simulink model "pruebaswitch2"  (R2016b)
settings: Solver=VariableStepAuto  StartTime=0.0  StopTime=10.0  RelTol=1e-3
undefined symbols (not defined in the file): LD
settings Model: Creator=Uxío  LastModifiedBy=Uxío

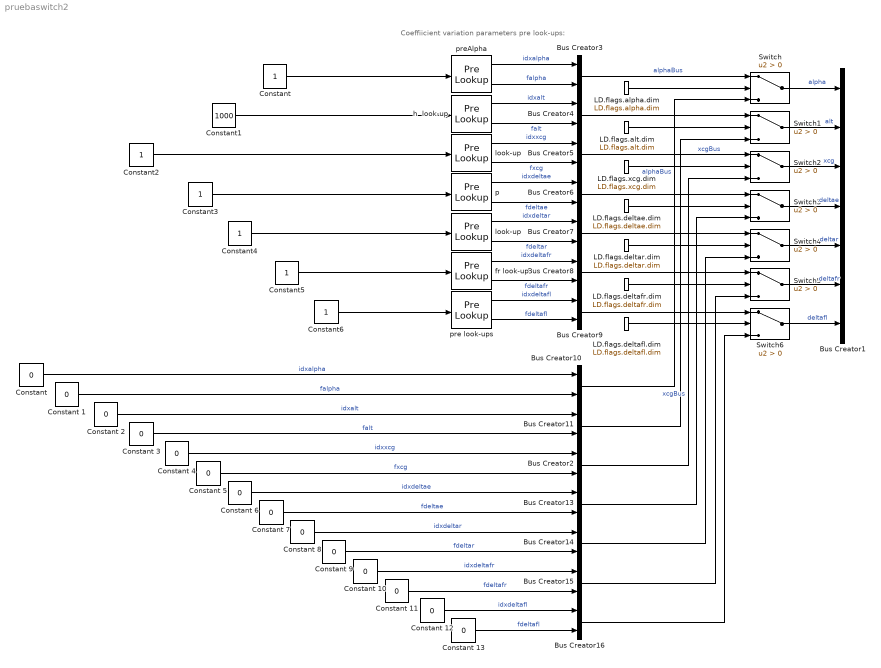
== system pruebaswitch2 ==
  note: Coeffiicient variation parameters pre look-ups:
  " look-up" : PreLookup  BreakpointsData=LD.xcg  BeginIndexSearchUsingPreviousIndexResult=on  IndexDataTypeStr=int32  FractionDataTypeStr=double
  Bus Creator1 : BusCreator  Inputs=7
  Bus Creator{2..11,13..16} (14 alike) : BusCreator  Inputs=2
  Constant{,2..6} (6 alike) : Constant
  Constant {,2,4,6,8,10,12} (7 alike) : Constant  Value=0  OutDataTypeStr=int32
  Constant {1,3,5,7,9,11,13} (7 alike) : Constant  Value=0
  Constant1 : Constant  Value=1000
  LD.flags.alpha.dim : Constant  Value=LD.flags.alpha.dim
  LD.flags.alt.dim : Constant  Value=LD.flags.alt.dim
  LD.flags.deltae.dim : Constant  Value=LD.flags.deltae.dim
  LD.flags.deltafl.dim : Constant  Value=LD.flags.deltafl.dim
  LD.flags.deltafr.dim : Constant  Value=LD.flags.deltafr.dim
  LD.flags.deltar.dim : Constant  Value=LD.flags.deltar.dim
  LD.flags.xcg.dim : Constant  Value=LD.flags.xcg.dim
  Switch{,1..6} (7 alike) : Switch  Criteria=u2 > Threshold
  fr look-up : PreLookup  BreakpointsData=LD.deltafr  BeginIndexSearchUsingPreviousIndexResult=on  IndexDataTypeStr=int32  FractionDataTypeStr=double
  h  look-up : PreLookup  BreakpointsData=LD.alt  BeginIndexSearchUsingPreviousIndexResult=on  IndexDataTypeStr=int32  FractionDataTypeStr=double
  look-up : PreLookup  BreakpointsData=LD.deltar  BeginIndexSearchUsingPreviousIndexResult=on  IndexDataTypeStr=int32  FractionDataTypeStr=double
  p : PreLookup  BreakpointsData=LD.deltae  BeginIndexSearchUsingPreviousIndexResult=on  IndexDataTypeStr=int32  FractionDataTypeStr=double
  pre look-ups : PreLookup  BreakpointsData=LD.deltafl  BeginIndexSearchUsingPreviousIndexResult=on  IndexDataTypeStr=int32  FractionDataTypeStr=double
  preAlpha : PreLookup  BreakpointsData=LD.alpha  BeginIndexSearchUsingPreviousIndexResult=on  IndexDataTypeStr=int32  FractionDataTypeStr=double
  wires:
  preAlpha/2 -> Bus Creator3/2  "falpha"
  preAlpha/1 -> Bus Creator3/1  "idxalpha"
  h  look-up/2 -> Bus Creator4/2  "falt"
  h  look-up/1 -> Bus Creator4/1  "idxalt"
  " look-up"/1 -> Bus Creator5/1  "idxxcg"
  " look-up"/2 -> Bus Creator5/2  "fxcg"
  p/2 -> Bus Creator6/2  "fdeltae"
  p/1 -> Bus Creator6/1  "idxdeltae"
  look-up/2 -> Bus Creator7/2  "fdeltar"
  look-up/1 -> Bus Creator7/1  "idxdeltar"
  fr look-up/2 -> Bus Creator8/2  "fdeltafr"
  fr look-up/1 -> Bus Creator8/1  "idxdeltafr"
  pre look-ups/1 -> Bus Creator9/1  "idxdeltafl"
  pre look-ups/2 -> Bus Creator9/2  "fdeltafl"
  Constant 1/1 -> Bus Creator10/2  "falpha"
  "Constant "/1 -> Bus Creator10/1  "idxalpha"
  Constant 3/1 -> Bus Creator11/2  "falt"
  Constant 2/1 -> Bus Creator11/1  "idxalt"
  Constant 4/1 -> Bus Creator2/1  "idxxcg"
  Constant 5/1 -> Bus Creator2/2  "fxcg"
  Constant 7/1 -> Bus Creator13/2  "fdeltae"
  Constant 6/1 -> Bus Creator13/1  "idxdeltae"
  Constant 9/1 -> Bus Creator14/2  "fdeltar"
  Constant 8/1 -> Bus Creator14/1  "idxdeltar"
  Constant 11/1 -> Bus Creator15/2  "fdeltafr"
  Constant 10/1 -> Bus Creator15/1  "idxdeltafr"
  Constant 12/1 -> Bus Creator16/1  "idxdeltafl"
  Constant 13/1 -> Bus Creator16/2  "fdeltafl"
  LD.flags.alpha.dim/1 -> Switch/2
  Bus Creator3/1 -> Switch/1  "alphaBus"
  LD.flags.alt.dim/1 -> Switch1/2
  Bus Creator4/1 -> Switch1/1
  LD.flags.xcg.dim/1 -> Switch2/2
  Bus Creator5/1 -> Switch2/1  "xcgBus"
  LD.flags.deltae.dim/1 -> Switch3/2
  Bus Creator6/1 -> Switch3/1
  LD.flags.deltar.dim/1 -> Switch4/2
  Bus Creator7/1 -> Switch4/1
  LD.flags.deltafr.dim/1 -> Switch5/2
  Bus Creator8/1 -> Switch5/1
  LD.flags.deltafl.dim/1 -> Switch6/2
  Bus Creator9/1 -> Switch6/1
  Bus Creator10/1 -> Switch/3  "alphaBus"
  Bus Creator11/1 -> Switch1/3
  Bus Creator2/1 -> Switch2/3  "xcgBus"
  Bus Creator13/1 -> Switch3/3
  Bus Creator14/1 -> Switch4/3
  Bus Creator15/1 -> Switch5/3
  Bus Creator16/1 -> Switch6/3
  Switch/1 -> Bus Creator1/1  "alpha"
  Switch1/1 -> Bus Creator1/2  "alt"
  Switch2/1 -> Bus Creator1/3  "xcg"
  Switch3/1 -> Bus Creator1/4  "deltae"
  Switch4/1 -> Bus Creator1/5  "deltar"
  Switch5/1 -> Bus Creator1/6  "deltafr"
  Switch6/1 -> Bus Creator1/7  "deltafl"
  Constant/1 -> preAlpha/1
  Constant1/1 -> h  look-up/1
  Constant2/1 -> " look-up"/1
  Constant3/1 -> p/1
  Constant4/1 -> look-up/1
  Constant5/1 -> fr look-up/1
  Constant6/1 -> pre look-ups/1
